simulink model "Ejemplo0313_simulink"  (R2024b)
settings: Solver=VariableStepAuto  StartTime=0.0  StopTime=500  RelTol=1e-3
values from neighbouring files (symbols this model uses):
  B = ceil(Kv_nuevo/Kv_original)    [Ejemplo0508_retraso.m]
  K = 1.91    [Ejemplo0409_lgr.m]    (also in Ejemplo0422_KhK.m = 0.156; Ejemplo0506_compensadoradelanto.m = 11; Ejemplo0508_retraso.m = 0.80:0.01:1.1; Ejemplo0527_criterionyquist.m = 1)
undefined symbols (not defined in the file or in its folder): J, Tr
settings Model: Creator=carlosjuarez  LastModifiedBy=carlosjuarez

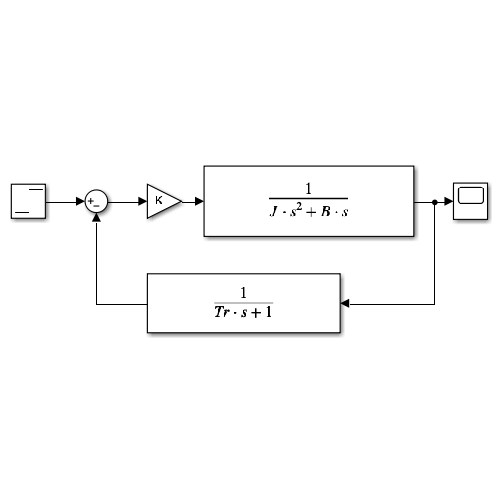
[thumbnail: Simulink's stored preview of the top-level diagram]
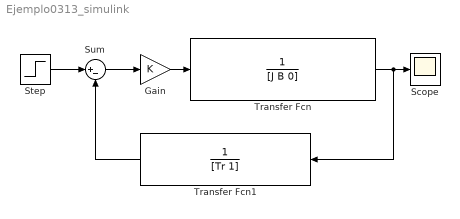
== system Ejemplo0313_simulink ==
  Gain : Gain  Gain=K
  Scope : Scope
  Step : Step  SampleTime=0
  Sum : Sum  Inputs=|+-
  Transfer Fcn : TransferFcn  Denominator=[J B 0]
  Transfer Fcn1 : TransferFcn  Denominator=[Tr 1]
  wires:
  Transfer Fcn/1 -> Transfer Fcn1/1, Scope/1
  Gain/1 -> Transfer Fcn/1
  Step/1 -> Sum/1
  Sum/1 -> Gain/1
  Transfer Fcn1/1 -> Sum/2
